simulink model "Example_Hydraulic_Thermosyphon"  (R2013b)
settings: Solver=ode45  StartTime=0.0  StopTime=3600  RelTol=1e-3
libraries: carnot x6
settings Model: Creator=drhf  LastModifiedBy=drhf
settings DataIOCC: SignalLoggingSaveFormat=ModelDataLogs
settings OptimizationCC: ExpressionDepthLimit=2147483647
settings DebuggingCC: FcnCallInpInsideContextMsg=EnableAllAsWarning  StateNameClashWarn=warning
settings GRTTargetCC: CombineOutputUpdateFcns=off  GRTInterface=on

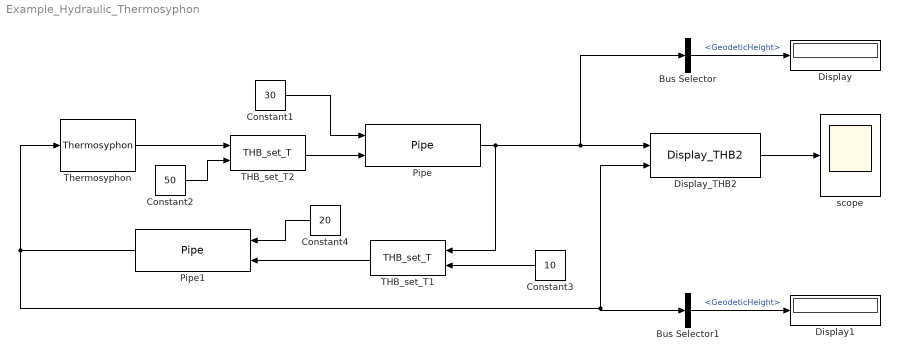
== system Example_Hydraulic_Thermosyphon ==
  Bus Selector : BusSelector  OutputSignals=GeodeticHeight
  Bus Selector1 : BusSelector  OutputSignals=GeodeticHeight
  Constant1 : Constant  Value=30
  Constant2 : Constant  Value=50
  Constant3 : Constant  Value=10
  Constant4 : Constant  Value=20
  Display : Display
  Display1 : Display
  Display_THB2 : carnot/Outputs/Display_THB2  t=off  m=on  p=off  id=off  mix=off  d=off
  Pipe : carnot/Hydraulics/Pipe  dia=0.02  len=10  hgt=5  uloss=100/20/10  cond=0  cwall=1000  t0=20  lin=100/0.2  qua=100/0.2^2  nodes=10
  Pipe1 : carnot/Hydraulics/Pipe  dia=0.02  len=10  hgt=-5  uloss=100/20/10  cond=0  cwall=1000  t0=20  lin=100/0.2  qua=100/0.2^2  nodes=10
  THB_set_T1 : carnot/Source/Simple/THB_set_T
  THB_set_T2 : carnot/Source/Simple/THB_set_T
  Thermosyphon : carnot/Hydraulics/Thermosyphon  dia=0.025  fluid_id=water  mix=0  p0=2e5  t1=5
  scope : Scope
      settings: TickLabels=on  YMin=0
  wires:
  Display_THB2/1 -> scope/1
  Pipe1/1 -> Bus Selector1/1, Display_THB2/2, Thermosyphon/1
  Thermosyphon/1 -> THB_set_T2/1
  THB_set_T2/1 -> Pipe/2
  Constant1/1 -> Pipe/1
  Constant2/1 -> THB_set_T2/2
  THB_set_T1/1 -> Pipe1/2
  Pipe/1 -> THB_set_T1/1, Display_THB2/1, Bus Selector/1
  Constant3/1 -> THB_set_T1/2
  Bus Selector/1 -> Display/1  "<GeodeticHeight>"
  Bus Selector1/1 -> Display1/1  "<GeodeticHeight>"
  Constant4/1 -> Pipe1/1
